simulink model "ZynqBallTrackerFPGA"  (R2017a)
settings: Solver=FixedStepDiscrete  StartTime=0.0  StopTime=5.0  RelTol=1e-3  EnableMultiTasking=on
PostLoadFcn:
  | model_init
values from neighbouring files (symbols this model uses):
  C = 1920    [model_init.m]
  HueTarg = 150    [model_init.m]
  HueTol = 20    [model_init.m]
  Kd = 1    [model_init.m]
  KernG_hdl = reshape(KernG,[],1)    [model_init.m]
  KernR1B2_hdl = reshape(KernR1B2,[],1)    [model_init.m]
  KernR2B1_hdl = reshape(KernR2B1,[],1)    [model_init.m]
  KernRB_hdl = reshape(KernRB,[],1)    [model_init.m]
  Ki = 4    [model_init.m]
  Kp = 16    [model_init.m]
  P = polyfit(u,y,N)    [calc_gamma.m]    (also in model_init.m = calc_gamma(GammaErr,3))
  PWM_CNT = 1024e3    (= 1024000)    [model_init.m]
  R = 1080    [model_init.m]
  SatTarg = 0.38    [model_init.m]
  SatTol = 0.05    [model_init.m]
  SaturationLimit = 256    [model_init.m]
  TsFPGA = TsFr/(R*C)    (= 1.60751028807e-08)    [model_init.m]
  TsFr = 1/FrRt    (= 0.0333333333333)    [model_init.m]
  ValTarg = 170    [model_init.m]
  ValTol = 45    [model_init.m]
undefined symbols (not defined in the file or in its folder): gray, Rec, SDTV
libraries: hdlsllib x51, simulink x12, simulink_need_slupdate x10, visionconversions x2, visiontextngfix x2, visionstatistics x1, dspvision x1, visiongeotforms x1, dspsigattribs x1, dspbuff3 x1
(part 2 of 2)

== system ZynqBallTrackerFPGA/fpga_dut/BallTracker/FindCentroid/y_accum ==
  Inc : Inport
  Rst : Inport  Port=2
  En : Inport  Port=3
  Add : Sum  OutDataTypeStr=fixdt(0,ceil(log2(MaxVal)),0)  RndMeth=Zero  SaturateOnIntegerOverflow=on
  Logical Operator : Logic  Operator=OR  IconShape=distinctive  AllPortsSameDT=off  OutDataTypeStr=boolean
  Switch : Switch  Criteria=u2 ~= 0
  Unit Delay Enabled : simulink_need_slupdate/Unit Delay Enabled  vinit=fi(0,0,32,0)  tsamp=-1
      settings: SourceProductName=Simulink  SourceProductBaseCode=SL
  zero : Constant  Value=0  OutDataTypeStr=Inherit: Inherit via back propagation  SampleTime=-1
  Cnt : Outport
  wires:
  En/1 -> Logical Operator/2
  Rst/1 -> Logical Operator/1, Switch/2
  zero/1 -> Switch/1
  Add/1 -> Switch/3
  Logical Operator/1 -> Unit Delay Enabled/2
  Switch/1 -> Unit Delay Enabled/1
  Inc/1 -> Add/2  "xinc"
  Unit Delay Enabled/1 -> Add/1, Cnt/1

== system ZynqBallTrackerFPGA/fpga_dut/BallTracker/OutputMux/HuetoRGB ==
  Hue : Inport
  Gain : Gain  Gain=255/360  OutDataTypeStr=fixdt(0,8,0)  RndMeth=Zero  SaturateOnIntegerOverflow=on
      settings: AttributesFormatString=|
      | ----------
      | op:3
      | ip:1
  Y2RGB : Subsystem
  RGB : Outport
  wires:
  Hue/1 -> Gain/1
  Gain/1 -> Y2RGB/1(Y_i)
  Y2RGB/1(Video_Out) -> RGB/1

== system ZynqBallTrackerFPGA/fpga_dut/BallTracker/OutputMux/SattoRGB2 ==
  Sat : Inport
  Gain : Gain  Gain=255  OutDataTypeStr=fixdt(0,8,0)  RndMeth=Zero  SaturateOnIntegerOverflow=on
      settings: AttributesFormatString=|
      | ----------
      | op:3
      | ip:1
  Y2RGB : Subsystem
  RGB : Outport
  wires:
  Sat/1 -> Gain/1
  Gain/1 -> Y2RGB/1(Y_i)
  Y2RGB/1(Video_Out) -> RGB/1

== system ZynqBallTrackerFPGA/fpga_dut/BallTracker/OutputMux/Y2RGB ==
  Y_i : Inport
  Bit Concat : hdlsllib/HDL Operations/Bit Concat  numInputs=2
      settings: SourceProductName=HDL Coder  SourceProductBaseCode=HD
  Bit Concat1 : hdlsllib/HDL Operations/Bit Concat  numInputs=2
      settings: SourceProductName=HDL Coder  SourceProductBaseCode=HD
  Bit Concat2 : hdlsllib/HDL Operations/Bit Concat  numInputs=2
      settings: SourceProductName=HDL Coder  SourceProductBaseCode=HD
  Constant : Constant  Value=0  OutDataTypeStr=uint8  SampleTime=-1
  Video_Out : Outport  OutMin=0  OutMax=255
  wires:
  Bit Concat2/1 -> Bit Concat1/2
  Y_i/1 -> Bit Concat2/2, Bit Concat2/1, Bit Concat1/1
  Bit Concat1/1 -> Bit Concat/2
  Constant/1 -> Bit Concat/1
  Bit Concat/1 -> Video_Out/1

== system ZynqBallTrackerFPGA/fpga_dut/BallTracker/OutputMux/Y2RGB1 ==
  Y_i : Inport
  Bit Concat : hdlsllib/HDL Operations/Bit Concat  numInputs=2
      settings: SourceProductName=HDL Coder  SourceProductBaseCode=HD
  Bit Concat1 : hdlsllib/HDL Operations/Bit Concat  numInputs=2
      settings: SourceProductName=HDL Coder  SourceProductBaseCode=HD
  Bit Concat2 : hdlsllib/HDL Operations/Bit Concat  numInputs=2
      settings: SourceProductName=HDL Coder  SourceProductBaseCode=HD
  Constant : Constant  Value=0  OutDataTypeStr=uint8  SampleTime=-1
  Video_Out : Outport  OutMin=0  OutMax=255
  wires:
  Bit Concat2/1 -> Bit Concat1/2
  Y_i/1 -> Bit Concat2/2, Bit Concat2/1, Bit Concat1/1
  Bit Concat1/1 -> Bit Concat/2
  Constant/1 -> Bit Concat/1
  Bit Concat/1 -> Video_Out/1

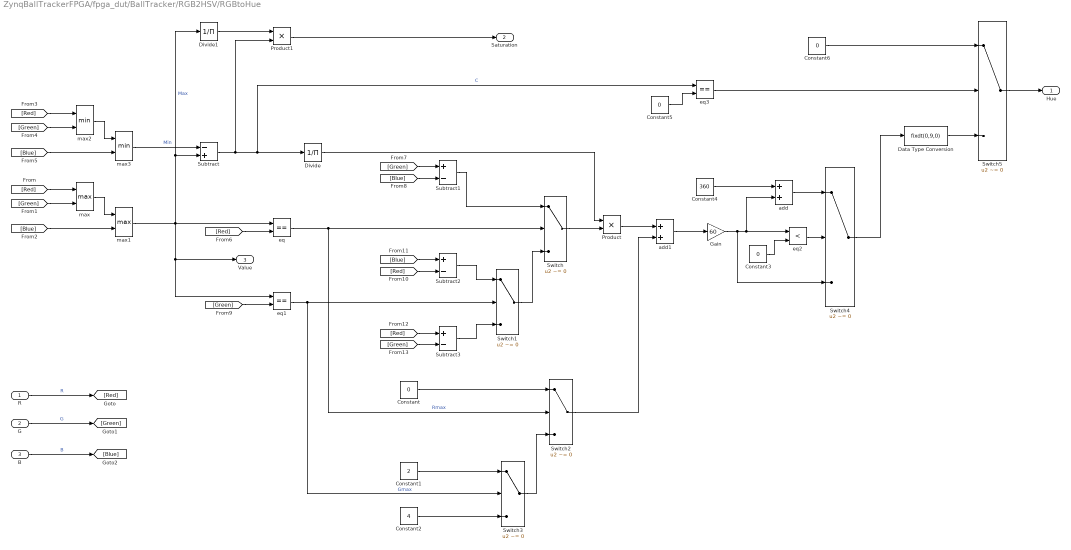
== system ZynqBallTrackerFPGA/fpga_dut/BallTracker/RGB2HSV/RGBtoHue ==
  R : Inport
  G : Inport  Port=2
  B : Inport  Port=3
  Constant : Constant  Value=0  OutDataTypeStr=fixdt(0,3,0)  SampleTime=-1
  Constant1 : Constant  Value=2  OutDataTypeStr=fixdt(0,3,0)  SampleTime=-1
  Constant2 : Constant  Value=4  OutDataTypeStr=fixdt(0,3,0)  SampleTime=-1
  Constant3 : Constant  Value=0  OutDataTypeStr=Inherit: Inherit via back propagation  SampleTime=-1
  Constant4 : Constant  Value=360  OutDataTypeStr=Inherit: Inherit via back propagation  SampleTime=-1
  Constant5 : Constant  Value=0  OutDataTypeStr=Inherit: Inherit via back propagation  SampleTime=-1
  Constant6 : Constant  Value=0  OutDataTypeStr=Inherit: Inherit via back propagation  SampleTime=-1
  Data Type Conversion : DataTypeConversion  OutDataTypeStr=fixdt(0,9,0)
  Divide : Product  Inputs=/  OutMin=1/255  OutMax=1  OutDataTypeStr=fixdt(1,16)  SaturateOnIntegerOverflow=on  RndMeth=Zero
      settings: AttributesFormatString=|
      | ----------
      | op:3
      | ip:1
  Divide1 : Product  Inputs=/  OutMin=1/255  OutMax=1  OutDataTypeStr=fixdt(0,16)  SaturateOnIntegerOverflow=on  RndMeth=Zero
      settings: AttributesFormatString=|
      | ----------
      | op:3
      | ip:1
  Gain : Gain  Gain=60  ParamDataTypeStr=fixdt(1,7)  OutDataTypeStr=fixdt(1,10,0)  RndMeth=Zero
      settings: AttributesFormatString=|
      | ----------
      | op:3
      | ip:1
  Product : Product
      settings: AttributesFormatString=|
      | ----------
      | op:3
      | ip:1
  Product1 : Product  OutDataTypeStr=fixdt(0,16,15)  SaturateOnIntegerOverflow=on  RndMeth=Zero
      settings: AttributesFormatString=|
      | ----------
      | op:3
      | ip:1
  Subtract : Sum  Inputs=-+  RndMeth=Zero  OutDataTypeStr=Inherit: Same as first input
      settings: AttributesFormatString=|
      | ----------
      | op:1
  Subtract1 : Sum  Inputs=+-  RndMeth=Zero
      settings: AttributesFormatString=|
      | ----------
      | op:1
  Subtract2 : Sum  Inputs=+-  RndMeth=Zero
      settings: AttributesFormatString=|
      | ----------
      | op:1
  Subtract3 : Sum  Inputs=+-  RndMeth=Zero
      settings: AttributesFormatString=|
      | ----------
      | op:1
  Switch{,1..5} (6 alike) : Switch  Criteria=u2 ~= 0
      settings: AttributesFormatString=|
      | ----------
      | op:1
      | ip:1
  add : Sum  OutDataTypeStr=Inherit: Inherit via back propagation  RndMeth=Zero
      settings: AttributesFormatString=|
      | ----------
      | op:1
  add1 : Sum  RndMeth=Zero  OutDataTypeStr=Inherit: Same as first input
      settings: AttributesFormatString=|
      | ----------
      | op:1
  eq : RelationalOperator  Operator===  OutDataTypeStr=boolean  RndMeth=Nearest
  eq1 : RelationalOperator  Operator===  OutDataTypeStr=boolean  RndMeth=Nearest
  eq2 : RelationalOperator  Operator=<  OutDataTypeStr=boolean  RndMeth=Nearest
  eq3 : RelationalOperator  Operator===  OutDataTypeStr=boolean  RndMeth=Nearest
  max : MinMax  Function=max  Inputs=2
  max1 : MinMax  Function=max  Inputs=2
  max2 : MinMax  Inputs=2
  max3 : MinMax  Inputs=2
  Hue : Outport
  Saturation : Outport  Port=2
  Value : Outport  Port=3
  wires:
  R/1 -> [Red]  "R"
  B/1 -> [Blue]  "B"
  G/1 -> [Green]  "G"
  [Red] -> max/1
  [Green] -> max/2
  max/1 -> max1/1
  [Blue] -> max1/2
  [Red] -> max2/1
  [Green] -> max2/2
  max2/1 -> max3/1
  [Blue] -> max3/2
  max1/1 -> eq/1, Value/1, eq1/1, Divide1/1, Subtract/2  "Max"
  max3/1 -> Subtract/1  "Min"
  [Red] -> eq/2
  [Blue] -> Subtract1/2
  [Green] -> Subtract1/1
  Switch1/1 -> Switch/3
  [Green] -> eq1/2
  eq1/1 -> Switch3/2, Switch1/2  "Gmax"
  [Blue] -> Subtract2/1
  [Red] -> Subtract2/2
  Subtract2/1 -> Switch1/1
  Subtract3/1 -> Switch1/3
  [Red] -> Subtract3/1
  [Green] -> Subtract3/2
  Subtract1/1 -> Switch/1
  Product/1 -> add1/1
  eq/1 -> Switch/2, Switch2/2  "Rmax"
  Switch/1 -> Product/2
  Subtract/1 -> Product1/2, eq3/1, Divide/1  "C"
  Divide/1 -> Product/1
  Switch3/1 -> Switch2/3
  Constant/1 -> Switch2/1
  Constant1/1 -> Switch3/1
  Constant2/1 -> Switch3/3
  Switch2/1 -> add1/2
  add1/1 -> Gain/1
  Gain/1 -> Switch4/3, add/2, eq2/1
  Constant3/1 -> eq2/2
  eq2/1 -> Switch4/2
  Constant4/1 -> add/1
  add/1 -> Switch4/1
  Constant5/1 -> eq3/2
  eq3/1 -> Switch5/2
  Switch5/1 -> Hue/1
  Switch4/1 -> Data Type Conversion/1
  Constant6/1 -> Switch5/1
  Data Type Conversion/1 -> Switch5/3
  Divide1/1 -> Product1/1
  Product1/1 -> Saturation/1

== system ZynqBallTrackerFPGA/fpga_dut/CFA/MW_CFA/Bayer_to_Vid ==
  SoF : Inport
  Bayer : Inport  Port=2
  Bit Concat{,1..3} (4 alike) : hdlsllib/HDL Operations/Bit Concat  numInputs=2
      settings: SourceProductName=HDL Coder  SourceProductBaseCode=HD
  Constant : Constant  Value=0  OutDataTypeStr=fixdt(0,7,0)  SampleTime=-1
  Video_o : Outport
  wires:
  Bit Concat1/1 -> Bit Concat3/2
  SoF/1 -> Bit Concat/1
  Bayer/1 -> Bit Concat1/1, Bit Concat2/1, Bit Concat2/2
  Bit Concat2/1 -> Bit Concat1/2
  Bit Concat/1 -> Video_o/1
  Constant/1 -> Bit Concat3/1
  Bit Concat3/1 -> Bit Concat/2

== system ZynqBallTrackerFPGA/fpga_dut/CFA/MW_CFA/Buff_5x5 ==
  Pixel : Inport
  Delay{1..4} (4 alike) : Delay  DelayLength=1  InitialCondition=0  UseCircularBuffer=on
  Integer Delay{1..4} (4 alike) : Delay  DelayLength=C
  Matrix Concatenation 25_1 : Concatenate  NumInputs=5  Mode=Multidimensional array
  Matrix Concatenation 5_1 : Concatenate  NumInputs=5  Mode=Multidimensional array
  Dly_5x5 : Outport
  wires:
  Delay2/1 -> Matrix Concatenation 25_1/2, Delay3/1
  Matrix Concatenation 5_1/1 -> Delay4/1, Matrix Concatenation 25_1/5
  Delay3/1 -> Matrix Concatenation 25_1/1
  Matrix Concatenation 25_1/1 -> Dly_5x5/1
  Delay1/1 -> Matrix Concatenation 25_1/3, Delay2/1
  Delay4/1 -> Delay1/1, Matrix Concatenation 25_1/4
  Pixel/1 -> Matrix Concatenation 5_1/5, Integer Delay1/1
  Integer Delay1/1 -> Matrix Concatenation 5_1/4, Integer Delay2/1
  Integer Delay2/1 -> Matrix Concatenation 5_1/3, Integer Delay3/1
  Integer Delay3/1 -> Matrix Concatenation 5_1/2, Integer Delay4/1
  Integer Delay4/1 -> Matrix Concatenation 5_1/1

== system ZynqBallTrackerFPGA/fpga_dut/CFA/MW_CFA/Calc_Kern ==
  Dly_5x5 : Inport
  KernG : Gain  Gain=KernG_hdl  ParamDataTypeStr=fixdt(1,8)
      settings: AttributesFormatString=|
      | ----------
      | op:3
      | ip:2
  KernR1B2 : Gain  Gain=KernR1B2_hdl  ParamDataTypeStr=fixdt(1,8)
      settings: AttributesFormatString=|
      | ----------
      | op:3
      | ip:2
  KernR2B1 : Gain  Gain=KernR2B1_hdl  ParamDataTypeStr=fixdt(1,8)
      settings: AttributesFormatString=|
      | ----------
      | op:3
      | ip:2
  KernRB : Gain  Gain=KernRB_hdl  ParamDataTypeStr=fixdt(1,8)
      settings: AttributesFormatString=|
      | ----------
      | op:3
      | ip:2
  SumG : Sum  Inputs=+  OutDataTypeStr=uint8  RndMeth=Zero  SaturateOnIntegerOverflow=on
      settings: AttributesFormatString=|
      | ----------
      | op:4
      | ip:2
  SumR1B2 : Sum  Inputs=+  OutDataTypeStr=uint8  RndMeth=Zero  SaturateOnIntegerOverflow=on
      settings: AttributesFormatString=|
      | ----------
      | op:4
      | ip:2
  SumR2B1 : Sum  Inputs=+  OutDataTypeStr=uint8  RndMeth=Zero  SaturateOnIntegerOverflow=on
      settings: AttributesFormatString=|
      | ----------
      | op:4
      | ip:2
  SumRB : Sum  Inputs=+  OutDataTypeStr=uint8  RndMeth=Zero  SaturateOnIntegerOverflow=on
      settings: AttributesFormatString=|
      | ----------
      | op:4
      | ip:2
  Ir1b2 : Outport
  Ir2b1 : Outport  Port=2
  Irb : Outport  Port=3
  Ig : Outport  Port=4
  wires:
  Dly_5x5/1 -> KernR1B2/1, KernR2B1/1, KernG/1, KernRB/1
  KernG/1 -> SumG/1
  SumR1B2/1 -> Ir1b2/1  "Ir1b2"
  SumR2B1/1 -> Ir2b1/1  "Ir2b1"
  KernRB/1 -> SumRB/1
  KernR2B1/1 -> SumR2B1/1
  SumG/1 -> Ig/1  "Ig"
  SumRB/1 -> Irb/1  "Irb"
  KernR1B2/1 -> SumR1B2/1

== system ZynqBallTrackerFPGA/fpga_dut/CFA/MW_CFA/RGB_to_Vid ==
  SoF : Inport
  R : Inport  Port=2
  G : Inport  Port=3
  B : Inport  Port=4
  Bit Concat{,1..3} (4 alike) : hdlsllib/HDL Operations/Bit Concat  numInputs=2
      settings: SourceProductName=HDL Coder  SourceProductBaseCode=HD
  Constant : Constant  Value=0  OutDataTypeStr=fixdt(0,7,0)  SampleTime=-1
  Video_o : Outport
  wires:
  Bit Concat1/1 -> Bit Concat3/2
  SoF/1 -> Bit Concat/1
  R/1 -> Bit Concat1/1
  B/1 -> Bit Concat2/2
  G/1 -> Bit Concat2/1
  Bit Concat2/1 -> Bit Concat1/2
  Bit Concat/1 -> Video_o/1
  Constant/1 -> Bit Concat3/1
  Bit Concat3/1 -> Bit Concat/2

== system ZynqBallTrackerFPGA/fpga_dut/CFA/MW_CFA/Select_Pixel ==
  note: State Encoding [RGGB]:
      | 	0 = Blue Pixel
      | 	1 = Green Pixel on blue row (1)
      | 	2 = Green Pixel on red row (2)
      | 	3 = Red Pixel
  I : Inport
  Ir1b2 : Inport  Port=2
  Ir2b1 : Inport  Port=3
  Irb : Inport  Port=4
  Ig : Inport  Port=5
  State : Inport  Port=6
  SelectBlue : Subsystem
  SelectGreen : Subsystem
  SelectRed : Subsystem
  R : Outport
  G : Outport  Port=2
  B : Outport  Port=3
  wires:
  SelectBlue/1(B) -> B/1
  SelectRed/1(R) -> R/1
  Ig/1 -> SelectGreen/2(Ig)
  I/1 -> SelectGreen/1(I), SelectBlue/1(I), SelectRed/1(I)
  Ir1b2/1 -> SelectBlue/2(Ir1b2), SelectRed/2(Ir1b2)
  State/1 -> SelectRed/5(State), SelectBlue/5(State), SelectGreen/3(State)
  Irb/1 -> SelectRed/4(Irb), SelectBlue/4(Irb)
  Ir2b1/1 -> SelectBlue/3(Ir2b1), SelectRed/3(Ir2b1)
  SelectGreen/1(G) -> G/1

== system ZynqBallTrackerFPGA/fpga_dut/CFA/MW_CFA/StateTracking ==
  Rst : Inport
  Bayer_Phase : Inport  Port=2
  Pix_Pos : Subsystem
  en : Constant  Value=true  SampleTime=-1
  state_xor : simulink/Logic and Bit Operations/Bitwise Operator  logicop=XOR  UseBitMask=off  NumInputPorts=2  BitMask=bin2dec('11011001')  BitMaskRealWorld=Stored Integer
      settings: AttributesFormatString=|
      | ----------
      | op:1
      | ip:1
  xy_to_state : Subsystem
  state : Outport
  wires:
  Rst/1 -> Pix_Pos/2(Rst)
  en/1 -> Pix_Pos/1(Vld)
  Pix_Pos/1(Column) -> xy_to_state/1(x)
  Pix_Pos/2(Row) -> xy_to_state/2(y)
  xy_to_state/1(state) -> state_xor/1
  state_xor/1 -> state/1
  Bayer_Phase/1 -> state_xor/2

== system ZynqBallTrackerFPGA/fpga_dut/CFA/MW_CFA/get_sof ==
  Video_i : Inport
  Bit Slice : hdlsllib/HDL Operations/Bit Slice  lidx=31  ridx=31
      settings: SourceProductName=HDL Coder  SourceProductBaseCode=HD
  Data Type Conversion : DataTypeConversion  OutDataTypeStr=boolean
  Delay1 : Delay  DelayLength=1
  Delay2 : Delay  DelayLength=1
  SoF : Outport
  Video_o : Outport  Port=2
  Rst : Outport  Port=3
  wires:
  Bit Slice/1 -> Data Type Conversion/1
  Video_i/1 -> Delay2/1, Bit Slice/1
  Data Type Conversion/1 -> Rst/1, Delay1/1
  Delay2/1 -> Video_o/1
  Delay1/1 -> SoF/1

== system ZynqBallTrackerFPGA/fpga_dut/GammaCorrection/Gama CorrectionCore/GammaApprox ==
  Y_i : Inport
  P : Inport  Port=2
  Data Type Conversion : DataTypeConversion  OutDataTypeStr=fixdt(0,8,8)  SaturateOnIntegerOverflow=on  RndMeth=Zero
      settings: AttributesFormatString=|
      | ----------
      | op:1
      | ip:1
  Demux : Demux
  Gain1 : Gain  Gain=256  OutDataTypeStr=fixdt(0,8,0)  RndMeth=Zero  SaturateOnIntegerOverflow=on
      settings: AttributesFormatString=|
      | ----------
      | op:1
      | ip:1
  Gain2 : Gain  Gain=1/256  OutDataTypeStr=fixdt(0,8,8)  RndMeth=Zero  SaturateOnIntegerOverflow=on
      settings: AttributesFormatString=|
      | ----------
      | op:1
      | ip:1
  Product : Product  OutDataTypeStr=fixdt(1,18,17)
      settings: AttributesFormatString=|
      | ----------
      | op:2
      | ip:1
  Product1 : Product  OutDataTypeStr=fixdt(1,18,17)  SaturateOnIntegerOverflow=on  RndMeth=Zero
      settings: AttributesFormatString=|
      | ----------
      | op:3
      | ip:1
  aDSP48E1 : Subsystem
  bDSP48E1 : Subsystem
  cDSP48E1 : Subsystem
  Y_o : Outport
  wires:
  Gain1/1 -> Y_o/1
  Y_i/1 -> Gain2/1
  P/1 -> Demux/1
  Demux/2 -> bDSP48E1/2(A)
  Demux/1 -> aDSP48E1/2(A)
  Product1/1 -> aDSP48E1/1(B)  "X3"
  Gain2/1 -> Product/1, Product/2, cDSP48E1/1(B), Product1/2  "X"
  Product/1 -> bDSP48E1/1(B), Product1/1  "X2"
  Demux/4 -> cDSP48E1/3(C)
  Demux/3 -> cDSP48E1/2(A)
  bDSP48E1/1(P) -> aDSP48E1/3(C)
  cDSP48E1/1(P) -> bDSP48E1/3(C)
  aDSP48E1/1(P) -> Data Type Conversion/1
  Data Type Conversion/1 -> Gain1/1

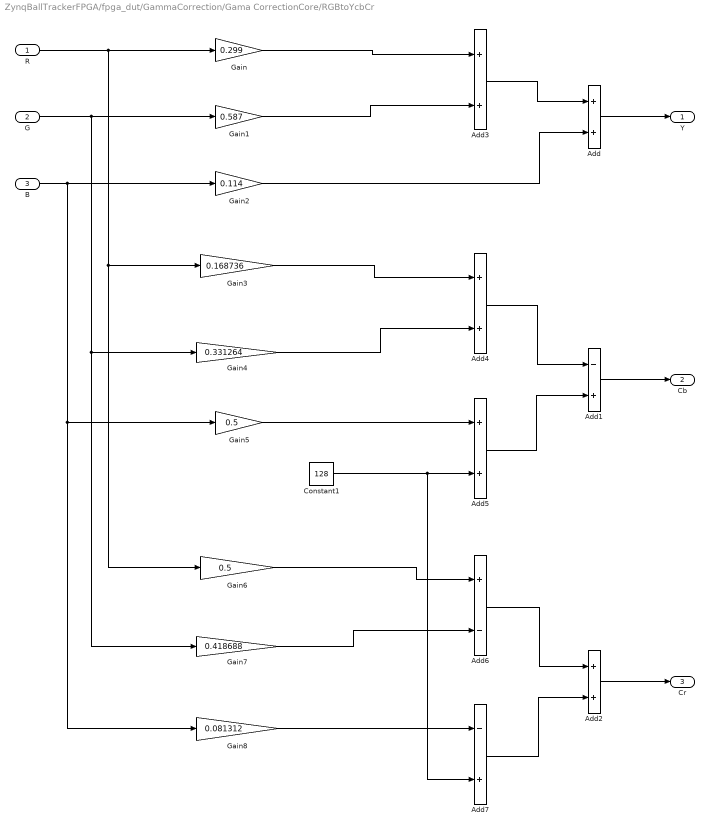
== system ZynqBallTrackerFPGA/fpga_dut/GammaCorrection/Gama CorrectionCore/RGBtoYcbCr ==
  R : Inport
  G : Inport  Port=2
  B : Inport  Port=3
  Add : Sum  OutDataTypeStr=uint8  RndMeth=Zero  SaturateOnIntegerOverflow=on
      settings: AttributesFormatString=|
      | ----------
      | op:2
      | ip:1
  Add1 : Sum  Inputs=-+  OutDataTypeStr=uint8  RndMeth=Zero  SaturateOnIntegerOverflow=on
      settings: AttributesFormatString=|
      | ----------
      | op:2
      | ip:1
  Add2 : Sum  OutDataTypeStr=uint8  RndMeth=Zero  SaturateOnIntegerOverflow=on
      settings: AttributesFormatString=|
      | ----------
      | op:2
      | ip:1
  Add3 : Sum  RndMeth=Zero  SaturateOnIntegerOverflow=on
      settings: AttributesFormatString=|
      | ----------
      | op:1
      | ip:1
  Add4 : Sum  RndMeth=Zero  SaturateOnIntegerOverflow=on
      settings: AttributesFormatString=|
      | ----------
      | op:1
      | ip:1
  Add5 : Sum  RndMeth=Zero  SaturateOnIntegerOverflow=on
      settings: AttributesFormatString=|
      | ----------
      | op:1
      | ip:1
  Add6 : Sum  Inputs=+-  RndMeth=Zero  SaturateOnIntegerOverflow=on
      settings: AttributesFormatString=|
      | ----------
      | op:1
      | ip:1
  Add7 : Sum  Inputs=-+  RndMeth=Zero  SaturateOnIntegerOverflow=on
      settings: AttributesFormatString=|
      | ----------
      | op:1
      | ip:1
  Constant1 : Constant  Value=128  OutDataTypeStr=fixdt(0,1)  SampleTime=-1
  Gain : Gain  Gain=0.299
      settings: AttributesFormatString=|
      | ----------
      | op:2
      | ip:1
  Gain1 : Gain  Gain=0.587
      settings: AttributesFormatString=|
      | ----------
      | op:2
      | ip:1
  Gain2 : Gain  Gain=0.114
      settings: AttributesFormatString=|
      | ----------
      | op:2
      | ip:1
  Gain3 : Gain  Gain=0.168736
      settings: AttributesFormatString=|
      | ----------
      | op:2
      | ip:1
  Gain4 : Gain  Gain=0.331264
      settings: AttributesFormatString=|
      | ----------
      | op:2
      | ip:1
  Gain5 : Gain  Gain=0.5
      settings: AttributesFormatString=|
      | ----------
      | op:2
      | ip:1
  Gain6 : Gain  Gain=0.5
      settings: AttributesFormatString=|
      | ----------
      | op:2
      | ip:1
  Gain7 : Gain  Gain=0.418688
      settings: AttributesFormatString=|
      | ----------
      | op:2
      | ip:1
  Gain8 : Gain  Gain=0.081312
      settings: AttributesFormatString=|
      | ----------
      | op:2
      | ip:1
  Y : Outport
  Cb : Outport  Port=2
  Cr : Outport  Port=3
  wires:
  G/1 -> Gain7/1, Gain4/1, Gain1/1
  Add/1 -> Y/1
  B/1 -> Gain8/1, Gain5/1, Gain2/1
  Constant1/1 -> Add7/2, Add5/2
  Gain3/1 -> Add4/1
  Gain5/1 -> Add5/1
  Add1/1 -> Cb/1
  R/1 -> Gain6/1, Gain3/1, Gain/1
  Gain4/1 -> Add4/2
  Gain6/1 -> Add6/1
  Gain8/1 -> Add7/1
  Add2/1 -> Cr/1
  Gain7/1 -> Add6/2
  Gain1/1 -> Add3/2
  Gain2/1 -> Add/2
  Gain/1 -> Add3/1
  Add3/1 -> Add/1
  Add4/1 -> Add1/1
  Add5/1 -> Add1/2
  Add6/1 -> Add2/1
  Add7/1 -> Add2/2

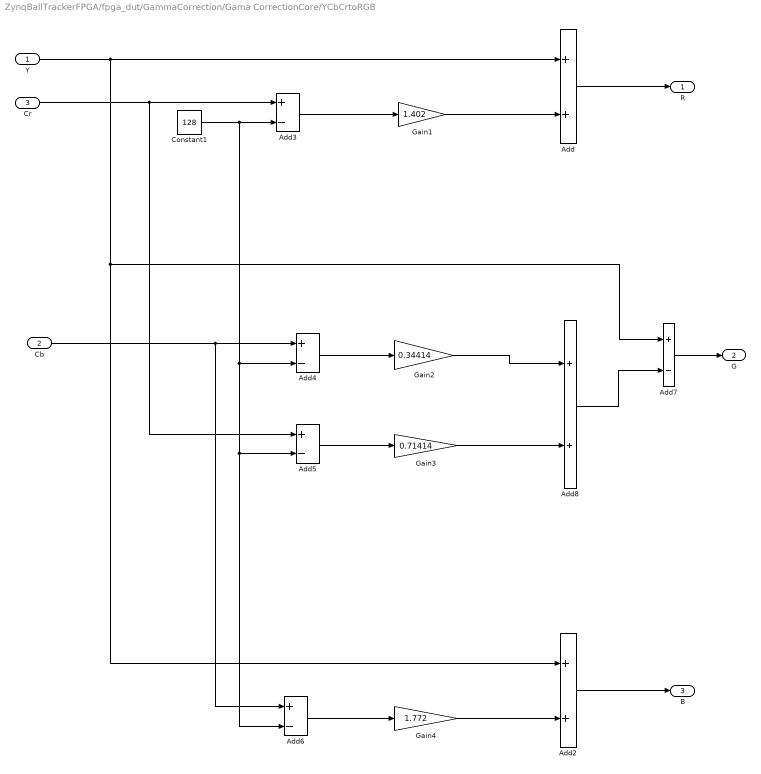
== system ZynqBallTrackerFPGA/fpga_dut/GammaCorrection/Gama CorrectionCore/YCbCrtoRGB ==
  Y : Inport
  Cb : Inport  Port=2
  Cr : Inport  Port=3
  Add : Sum  Inputs=2  OutDataTypeStr=uint8  RndMeth=Zero  SaturateOnIntegerOverflow=on
      settings: AttributesFormatString=|
      | ----------
      | op:2
      | ip:1
  Add2 : Sum  Inputs=2  OutDataTypeStr=uint8  RndMeth=Zero  SaturateOnIntegerOverflow=on
      settings: AttributesFormatString=|
      | ----------
      | op:2
      | ip:1
  Add{3..6} (4 alike) : Sum  Inputs=+-  RndMeth=Zero
      settings: AttributesFormatString=|
      | ----------
      | op:1
      | ip:1
  Add7 : Sum  Inputs=+-  OutDataTypeStr=uint8  RndMeth=Zero  SaturateOnIntegerOverflow=on
      settings: AttributesFormatString=|
      | ----------
      | op:2
      | ip:1
  Add8 : Sum  RndMeth=Zero  SaturateOnIntegerOverflow=on
      settings: AttributesFormatString=|
      | ----------
      | op:1
      | ip:1
  Constant1 : Constant  Value=128  OutDataTypeStr=fixdt(0,1)  SampleTime=-1
  Gain1 : Gain  Gain=1.402
      settings: AttributesFormatString=|
      | ----------
      | op:2
      | ip:1
  Gain2 : Gain  Gain=0.34414
      settings: AttributesFormatString=|
      | ----------
      | op:2
      | ip:1
  Gain3 : Gain  Gain=0.71414
      settings: AttributesFormatString=|
      | ----------
      | op:2
      | ip:1
  Gain4 : Gain  Gain=1.772
      settings: AttributesFormatString=|
      | ----------
      | op:2
      | ip:1
  R : Outport
  G : Outport  Port=2
  B : Outport  Port=3
  wires:
  Y/1 -> Add7/1, Add2/1, Add/1
  Add/1 -> R/1
  Cr/1 -> Add5/1, Add3/1
  Constant1/1 -> Add6/2, Add5/2, Add4/2, Add3/2
  Add3/1 -> Gain1/1
  Gain1/1 -> Add/2
  Gain3/1 -> Add8/2
  Gain2/1 -> Add8/1
  Add4/1 -> Gain2/1
  Add5/1 -> Gain3/1
  Cb/1 -> Add6/1, Add4/1
  Add2/1 -> B/1
  Add6/1 -> Gain4/1
  Gain4/1 -> Add2/2
  Add7/1 -> G/1
  Add8/1 -> Add7/2

== system ZynqBallTrackerFPGA/fpga_dut/motor_ctl/ADC_DUT/Debounce ==
  In : Inport
  Chart : Stateflow chart  TreatAsAtomicUnit=on
  Constant : Constant  Value=debounce_count  OutDataTypeStr=uint8  SampleTime=-1
  Out : Outport
  wires:
  Constant/1 -> Chart/2(count_debounce)
  Chart/1(y) -> Out/1
  In/1 -> Chart/1(u)

== system ZynqBallTrackerFPGA/fpga_dut/motor_ctl/ADC_DUT/reduce_8_to_4 ==
  In1 : Inport
  Bit Concat : hdlsllib/HDL Operations/Bit Concat  numInputs=4
      settings: SourceProductName=HDL Coder  SourceProductBaseCode=HD
  Bit Slice : hdlsllib/HDL Operations/Bit Slice  lidx=1  ridx=1
      settings: SourceProductName=HDL Coder  SourceProductBaseCode=HD
  Bit Slice1 : hdlsllib/HDL Operations/Bit Slice  lidx=3  ridx=3
      settings: SourceProductName=HDL Coder  SourceProductBaseCode=HD
  Bit Slice2 : hdlsllib/HDL Operations/Bit Slice  lidx=5  ridx=5
      settings: SourceProductName=HDL Coder  SourceProductBaseCode=HD
  Bit Slice3 : hdlsllib/HDL Operations/Bit Slice  lidx=7  ridx=7
      settings: SourceProductName=HDL Coder  SourceProductBaseCode=HD
  Out1 : Outport
  wires:
  Bit Slice/1 -> Bit Concat/4
  Bit Slice1/1 -> Bit Concat/3
  Bit Slice2/1 -> Bit Concat/2
  Bit Slice3/1 -> Bit Concat/1
  Bit Concat/1 -> Out1/1
  In1/1 -> Bit Slice2/1, Bit Slice1/1, Bit Slice/1, Bit Slice3/1

== system ZynqBallTrackerFPGA/fpga_dut/motor_ctl/PID_Controller/PID_Controller_Programmable ==
  error_delta : Inport
  PGain : Inport  Port=2  LockScale=on
  IGain : Inport  Port=3
  DGain : Inport  Port=4  LockScale=on
  Controller : Subsystem  MinMaxOverflowLogging=MinMaxAndOverflow
  InputRegister{1..4} (4 alike) : Delay  DelayLength=1  InputProcessing=Inherited
  OutputRegister1 : Delay  DelayLength=1  InputProcessing=Inherited
  controlsignal : Outport
  wires:
  OutputRegister1/1 -> controlsignal/1
  InputRegister1/1 -> Controller/1(error_delta)
  InputRegister3/1 -> Controller/4(Dgain)
  InputRegister2/1 -> Controller/2(Pgain)
  IGain/1 -> InputRegister4/1  "sdo_igain"
  DGain/1 -> InputRegister3/1  "sdo_dgain"
  PGain/1 -> InputRegister2/1  "sdo_pgain"
  error_delta/1 -> InputRegister1/1
  Controller/1(controlsignal) -> OutputRegister1/1
  InputRegister4/1 -> Controller/3(Igain)

== system ZynqBallTrackerFPGA/fpga_dut/motor_ctl/pwm_controller/pwm_bist ==
  drive_p_in : Inport
  drive_n_in : Inport  Port=2
  force_p : Inport  Port=3
  force_n : Inport  Port=4
  disable : Inport  Port=5
  Logical Operator1 : Logic  Operator=NOT  IconShape=distinctive  AllPortsSameDT=off  OutDataTypeStr=boolean
  Logical Operator{3,7,9..10} (4 alike) : Logic  Inputs=3  IconShape=distinctive  AllPortsSameDT=off  OutDataTypeStr=boolean
  Logical Operator2 : Logic  Operator=OR  IconShape=distinctive  AllPortsSameDT=off  OutDataTypeStr=boolean
  Logical Operator4 : Logic  Operator=NAND  Inputs=3  IconShape=distinctive  AllPortsSameDT=off  OutDataTypeStr=boolean
  Logical Operator5 : Logic  Operator=OR  IconShape=distinctive  AllPortsSameDT=off  OutDataTypeStr=boolean
  Logical Operator6 : Logic  Operator=NOT  IconShape=distinctive  AllPortsSameDT=off  OutDataTypeStr=boolean
  Logical Operator8 : Logic  Operator=NOT  IconShape=distinctive  AllPortsSameDT=off  OutDataTypeStr=boolean
  drive_p_out : Outport
  drive_n_out : Outport  Port=2
  reset_cntr : Outport  Port=3
  wires:
  disable/1 -> Logical Operator1/1
  Logical Operator4/1 -> reset_cntr/1
  Logical Operator1/1 -> Logical Operator3/2, Logical Operator7/2, Logical Operator10/3, Logical Operator9/3, Logical Operator4/3
  force_n/1 -> Logical Operator3/3, Logical Operator8/1
  force_p/1 -> Logical Operator7/3, Logical Operator6/1
  Logical Operator10/1 -> Logical Operator5/1
  Logical Operator9/1 -> Logical Operator2/1
  Logical Operator7/1 -> Logical Operator2/2
  Logical Operator3/1 -> Logical Operator5/2
  Logical Operator2/1 -> drive_p_out/1
  Logical Operator5/1 -> drive_n_out/1
  drive_p_in/1 -> Logical Operator9/1
  drive_n_in/1 -> Logical Operator10/1
  Logical Operator6/1 -> Logical Operator4/1, Logical Operator10/2, Logical Operator3/1
  Logical Operator8/1 -> Logical Operator4/2, Logical Operator9/2, Logical Operator7/1

== system ZynqBallTrackerFPGA/fpga_dut/motor_ctl/pwm_controller/pwm_logic ==
  note: At the end of every period
      | latch the value for duty-cycle
      | and the direction
  inref : Inport
  polarity : Inport  Port=2
  reset : Inport  Port=3
  pwm_cnt : Inport  Port=4
  Bit Shift : hdlsllib/HDL Operations/Bit Shift  mode=Shift Right Arithmetic  N=8
      settings: SourceProductName=HDL Coder  SourceProductBaseCode=HD
  HDL Counter : hdlsllib/HDL Operations/HDL Counter  CountType=Free running  CountInit=0  CountStep=1  CountMax=10e5  CountFromType=Initial value  CountFrom=0  CountResetPort=on  CountLoadPort=off  CountEnbPort=off  CountDirPort=off  CountDataType=Unsigned  CountWordLen=22  CountFracLen=0  CountSampTime=-1
      settings: SourceProductName=HDL Coder  SourceProductBaseCode=HD
  Logical Operator : Logic  Inputs=3  IconShape=distinctive  AllPortsSameDT=off  OutDataTypeStr=boolean
  Logical Operator1 : Logic  Inputs=3  IconShape=distinctive  AllPortsSameDT=off  OutDataTypeStr=boolean
  Logical Operator2 : Logic  Operator=NOT  IconShape=distinctive  AllPortsSameDT=off  OutDataTypeStr=boolean
  Logical Operator3 : Logic  Operator=NOT  IconShape=distinctive  AllPortsSameDT=off  OutDataTypeStr=boolean
  Logical Operator4 : Logic  Operator=OR  IconShape=distinctive  AllPortsSameDT=off  OutDataTypeStr=boolean
  Product : Product
  Relational Operator : RelationalOperator  Operator=<  OutDataTypeStr=boolean  RndMeth=Nearest
  Relational Operator1 : RelationalOperator  OutDataTypeStr=boolean  RndMeth=Nearest
  Unit Delay Enabled : simulink_need_slupdate/Unit Delay Enabled  vinit=0.0  tsamp=-1
      settings: SourceProductName=Simulink  SourceProductBaseCode=SL
  Unit Delay Enabled1 : simulink_need_slupdate/Unit Delay Enabled  vinit=0.0  tsamp=-1
      settings: SourceProductName=Simulink  SourceProductBaseCode=SL
  drive_p : Outport
  drive_n : Outport  Port=2
  pwm_trig : Outport  Port=3
  wires:
  Unit Delay Enabled1/1 -> Logical Operator/2, Logical Operator3/1
  reset/1 -> Logical Operator2/1, Logical Operator4/1
  Logical Operator2/1 -> Logical Operator1/3, Logical Operator/3
  Relational Operator1/1 -> pwm_trig/1, Unit Delay Enabled1/2, Logical Operator4/2, Unit Delay Enabled/2
  polarity/1 -> Unit Delay Enabled1/1
  Logical Operator1/1 -> drive_n/1
  inref/1 -> Unit Delay Enabled/1
  Logical Operator/1 -> drive_p/1
  Relational Operator/1 -> Logical Operator1/1, Logical Operator/1
  HDL Counter/1 -> Relational Operator1/1, Relational Operator/1
  Unit Delay Enabled/1 -> Product/1
  Product/1 -> Relational Operator/2
  pwm_cnt/1 -> Relational Operator1/2, Bit Shift/1
  Logical Operator4/1 -> HDL Counter/1
  Bit Shift/1 -> Product/2
  Logical Operator3/1 -> Logical Operator1/2

== system ZynqBallTrackerFPGA/fpga_dut/BallTracker/FindCentroid/TimingSubsystem/Pix_Pos ==
  Vld : Inport
  Rst : Inport  Port=2
  ColLimit : simulink/Logic and Bit Operations/Compare To Constant  relop===  const=C-1  OutDataTypeStr=boolean
  ColumnCntr : hdlsllib/HDL Operations/HDL Counter  CountType=Count limited  CountInit=0  CountStep=1  CountMax=C-1  CountFromType=Initial value  CountFrom=0  CountResetPort=on  CountLoadPort=off  CountEnbPort=on  CountDirPort=off  CountDataType=Unsigned  CountWordLen=ceil(log2(C))  CountFracLen=0  CountSampTime=1
      settings: SourceProductName=HDL Coder  SourceProductBaseCode=HD
  Logical Operator : Logic  AllPortsSameDT=off  OutDataTypeStr=boolean
  RowCntr : hdlsllib/HDL Operations/HDL Counter  CountType=Count limited  CountInit=0  CountStep=1  CountMax=R-1  CountFromType=Initial value  CountFrom=0  CountResetPort=on  CountLoadPort=off  CountEnbPort=on  CountDirPort=off  CountDataType=Unsigned  CountWordLen=ceil(log2(R))  CountFracLen=0  CountSampTime=1
      settings: SourceProductName=HDL Coder  SourceProductBaseCode=HD
  Column : Outport
  Row : Outport  Port=2
  wires:
  Vld/1 -> Logical Operator/2, ColumnCntr/2  "enable"
  ColumnCntr/1 -> Column/1, ColLimit/1  "column"
  RowCntr/1 -> Row/1  "row"
  ColLimit/1 -> Logical Operator/1  "new_row"
  Rst/1 -> RowCntr/1, ColumnCntr/1  "rst"
  Logical Operator/1 -> RowCntr/2

== system ZynqBallTrackerFPGA/fpga_dut/BallTracker/OutputMux/HuetoRGB/Y2RGB ==
  Y_i : Inport
  Bit Concat : hdlsllib/HDL Operations/Bit Concat  numInputs=2
      settings: SourceProductName=HDL Coder  SourceProductBaseCode=HD
  Bit Concat1 : hdlsllib/HDL Operations/Bit Concat  numInputs=2
      settings: SourceProductName=HDL Coder  SourceProductBaseCode=HD
  Bit Concat2 : hdlsllib/HDL Operations/Bit Concat  numInputs=2
      settings: SourceProductName=HDL Coder  SourceProductBaseCode=HD
  Constant : Constant  Value=0  OutDataTypeStr=uint8  SampleTime=-1
  Video_Out : Outport  OutMin=0  OutMax=255
  wires:
  Bit Concat/1 -> Video_Out/1
  Constant/1 -> Bit Concat/1
  Bit Concat1/1 -> Bit Concat/2
  Y_i/1 -> Bit Concat1/1, Bit Concat2/1, Bit Concat2/2
  Bit Concat2/1 -> Bit Concat1/2

== system ZynqBallTrackerFPGA/fpga_dut/BallTracker/OutputMux/SattoRGB2/Y2RGB ==
  Y_i : Inport
  Bit Concat : hdlsllib/HDL Operations/Bit Concat  numInputs=2
      settings: SourceProductName=HDL Coder  SourceProductBaseCode=HD
  Bit Concat1 : hdlsllib/HDL Operations/Bit Concat  numInputs=2
      settings: SourceProductName=HDL Coder  SourceProductBaseCode=HD
  Bit Concat2 : hdlsllib/HDL Operations/Bit Concat  numInputs=2
      settings: SourceProductName=HDL Coder  SourceProductBaseCode=HD
  Constant : Constant  Value=0  OutDataTypeStr=uint8  SampleTime=-1
  Video_Out : Outport  OutMin=0  OutMax=255
  wires:
  Bit Concat/1 -> Video_Out/1
  Constant/1 -> Bit Concat/1
  Bit Concat1/1 -> Bit Concat/2
  Y_i/1 -> Bit Concat1/1, Bit Concat2/1, Bit Concat2/2
  Bit Concat2/1 -> Bit Concat1/2

== system ZynqBallTrackerFPGA/fpga_dut/CFA/MW_CFA/Select_Pixel/SelectBlue ==
  I : Inport
  Ir1b2 : Inport  Port=2
  Ir2b1 : Inport  Port=3
  Irb : Inport  Port=4
  State : Inport  Port=5
  Multiport Switch : MultiPortSwitch  DataPortOrder=Zero-based contiguous  Inputs=4
      settings: AttributesFormatString=|
      | ----------
      | op:1
      | ip:1
  B : Outport
  wires:
  Multiport Switch/1 -> B/1  "blue"
  State/1 -> Multiport Switch/1
  Irb/1 -> Multiport Switch/5
  I/1 -> Multiport Switch/2
  Ir1b2/1 -> Multiport Switch/4
  Ir2b1/1 -> Multiport Switch/3

== system ZynqBallTrackerFPGA/fpga_dut/CFA/MW_CFA/Select_Pixel/SelectGreen ==
  I : Inport
  Ig : Inport  Port=2
  State : Inport  Port=3
  Multiport Switch : MultiPortSwitch  DataPortOrder=Zero-based contiguous  Inputs=4
      settings: AttributesFormatString=|
      | ----------
      | op:1
      | ip:1
  G : Outport
  wires:
  I/1 -> Multiport Switch/3, Multiport Switch/4
  Ig/1 -> Multiport Switch/5, Multiport Switch/2
  Multiport Switch/1 -> G/1  "green"
  State/1 -> Multiport Switch/1

== system ZynqBallTrackerFPGA/fpga_dut/CFA/MW_CFA/Select_Pixel/SelectRed ==
  I : Inport
  Ir1b2 : Inport  Port=2
  Ir2b1 : Inport  Port=3
  Irb : Inport  Port=4
  State : Inport  Port=5
  Multiport Switch : MultiPortSwitch  DataPortOrder=Zero-based contiguous  Inputs=4
      settings: AttributesFormatString=|
      | ----------
      | op:1
      | ip:1
  R : Outport
  wires:
  State/1 -> Multiport Switch/1
  Multiport Switch/1 -> R/1  "red"
  I/1 -> Multiport Switch/5
  Irb/1 -> Multiport Switch/2
  Ir2b1/1 -> Multiport Switch/4
  Ir1b2/1 -> Multiport Switch/3

== system ZynqBallTrackerFPGA/fpga_dut/CFA/MW_CFA/StateTracking/Pix_Pos ==
  Vld : Inport
  Rst : Inport  Port=2
  ColLimit : simulink/Logic and Bit Operations/Compare To Constant  relop===  const=C-1  OutDataTypeStr=boolean
  ColumnCntr : hdlsllib/HDL Operations/HDL Counter  CountType=Count limited  CountInit=0  CountStep=1  CountMax=C-1  CountFromType=Initial value  CountFrom=0  CountResetPort=on  CountLoadPort=off  CountEnbPort=on  CountDirPort=off  CountDataType=Unsigned  CountWordLen=ceil(log2(C))  CountFracLen=0  CountSampTime=1
      settings: SourceProductName=HDL Coder  SourceProductBaseCode=HD
  Logical Operator : Logic  AllPortsSameDT=off  OutDataTypeStr=boolean
  RowCntr : hdlsllib/HDL Operations/HDL Counter  CountType=Count limited  CountInit=0  CountStep=1  CountMax=R-1  CountFromType=Initial value  CountFrom=0  CountResetPort=on  CountLoadPort=off  CountEnbPort=on  CountDirPort=off  CountDataType=Unsigned  CountWordLen=ceil(log2(R))  CountFracLen=0  CountSampTime=1
      settings: SourceProductName=HDL Coder  SourceProductBaseCode=HD
  Column : Outport
  Row : Outport  Port=2
  wires:
  Vld/1 -> Logical Operator/2, ColumnCntr/2  "enable"
  ColumnCntr/1 -> Column/1, ColLimit/1  "column"
  RowCntr/1 -> Row/1  "row"
  ColLimit/1 -> Logical Operator/1  "new_row"
  Rst/1 -> RowCntr/1, ColumnCntr/1  "rst"
  Logical Operator/1 -> RowCntr/2

== system ZynqBallTrackerFPGA/fpga_dut/CFA/MW_CFA/StateTracking/xy_to_state ==
  x : Inport
  y : Inport  Port=2
  Bit Concat : hdlsllib/HDL Operations/Bit Concat  numInputs=2
      settings: SourceProductName=HDL Coder  SourceProductBaseCode=HD
  GetLSB_x : hdlsllib/HDL Operations/Bit Slice  lidx=0  ridx=0
      settings: SourceProductName=HDL Coder  SourceProductBaseCode=HD
  GetLSB_y : hdlsllib/HDL Operations/Bit Slice  lidx=0  ridx=0
      settings: SourceProductName=HDL Coder  SourceProductBaseCode=HD
  state : Outport
  wires:
  x/1 -> GetLSB_x/1
  y/1 -> GetLSB_y/1
  Bit Concat/1 -> state/1
  GetLSB_x/1 -> Bit Concat/2
  GetLSB_y/1 -> Bit Concat/1

== system ZynqBallTrackerFPGA/fpga_dut/GammaCorrection/Gama CorrectionCore/GammaApprox/aDSP48E1 ==
  note: Implements P = B*A + C
      | 	B = 18-bit input
      | 	A = 25-bit input
      | 	C = 48-bit input
      |
      | Consumes pipeline registers of DSP48E1
  B : Inport
  A : Inport  Port=2
  C : Inport  Port=3
  adder : Sum  RndMeth=Zero
      settings: AttributesFormatString=|
      | ----------
      | op:1
      | ip:1
  mult : Product
      settings: AttributesFormatString=|
      | ----------
      | ip:1
  P : Outport
  wires:
  A/1 -> mult/2  "a"
  B/1 -> mult/1  "b"
  C/1 -> adder/2  "c_in"
  adder/1 -> P/1  "p"
  mult/1 -> adder/1  "m"

== system ZynqBallTrackerFPGA/fpga_dut/GammaCorrection/Gama CorrectionCore/GammaApprox/bDSP48E1 ==
  note: Implements P = B*A + C
      | 	B = 18-bit input
      | 	A = 25-bit input
      | 	C = 48-bit input
      |
      | Consumes pipeline registers of DSP48E1
  B : Inport
  A : Inport  Port=2
  C : Inport  Port=3
  adder : Sum  RndMeth=Zero
      settings: AttributesFormatString=|
      | ----------
      | op:1
      | ip:1
  mult : Product
      settings: AttributesFormatString=|
      | ----------
      | ip:1
  P : Outport
  wires:
  mult/1 -> adder/1  "m"
  adder/1 -> P/1  "p"
  C/1 -> adder/2  "c_in"
  B/1 -> mult/1  "b"
  A/1 -> mult/2  "a"

== system ZynqBallTrackerFPGA/fpga_dut/GammaCorrection/Gama CorrectionCore/GammaApprox/cDSP48E1 ==
  note: Implements P = B*A + C
      | 	B = 18-bit input
      | 	A = 25-bit input
      | 	C = 48-bit input
      |
      | Consumes pipeline registers of DSP48E1
  B : Inport
  A : Inport  Port=2
  C : Inport  Port=3
  adder : Sum  RndMeth=Zero
      settings: AttributesFormatString=|
      | ----------
      | op:1
      | ip:1
  mult : Product
      settings: AttributesFormatString=|
      | ----------
      | ip:1
  P : Outport
  wires:
  A/1 -> mult/2  "a"
  B/1 -> mult/1  "b"
  C/1 -> adder/2  "c_in"
  adder/1 -> P/1  "p"
  mult/1 -> adder/1  "m"

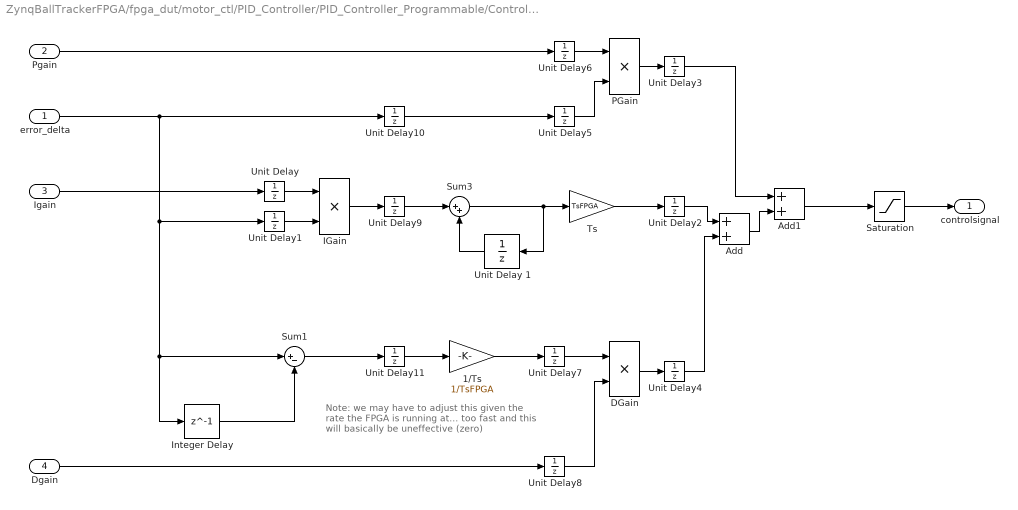
== system ZynqBallTrackerFPGA/fpga_dut/motor_ctl/PID_Controller/PID_Controller_Programmable/Controller ==
  note: Note: we may have to adjust this given
      | the rate the FPGA is running at... too fast
      | and this will basically be uneffective (zero)
  error_delta : Inport
  Pgain : Inport  Port=2
  Igain : Inport  Port=3
  Dgain : Inport  Port=4
  1/Ts : Gain  Gain=1/TsFPGA  SaturateOnIntegerOverflow=on
  Add : Sum
  Add1 : Sum
  DGain : Product  OutDataTypeStr=fixdt(1,24,0)
  IGain : Product
  Integer Delay : Delay  DelayLength=1  InputProcessing=Inherited
  PGain : Product
  Saturation : Saturate  UpperLimit=SaturationLimit-1  LowerLimit=-SaturationLimit  OutDataTypeStr=fixdt(1,9,0)
  Sum1 : Sum  Inputs=|+-  AccumDataTypeStr=fixdt(1,16,0)
  Sum3 : Sum  Inputs=|++  AccumDataTypeStr=fixdt(1,10,0)  OutDataTypeStr=fixdt(1,16,0)
  Ts : Gain  Gain=TsFPGA  SaturateOnIntegerOverflow=on
  Unit Delay{,1..11} (12 alike) : UnitDelay  SampleTime=-1
  Unit Delay 1 : UnitDelay  SampleTime=-1
  controlsignal : Outport
  wires:
  Saturation/1 -> controlsignal/1
  Dgain/1 -> Unit Delay8/1
  Pgain/1 -> Unit Delay6/1
  PGain/1 -> Unit Delay3/1
  1/Ts/1 -> Unit Delay7/1
  Sum1/1 -> Unit Delay11/1
  Integer Delay/1 -> Sum1/2
  error_delta/1 -> Unit Delay1/1, Integer Delay/1, Sum1/1, Unit Delay10/1
  DGain/1 -> Unit Delay4/1
  Sum3/1 -> Ts/1, Unit Delay 1/1
  Unit Delay 1/1 -> Sum3/2
  Igain/1 -> Unit Delay/1
  Unit Delay/1 -> IGain/1
  Unit Delay1/1 -> IGain/2
  Unit Delay2/1 -> Add/1
  Unit Delay3/1 -> Add1/1
  Unit Delay4/1 -> Add/2
  Unit Delay5/1 -> PGain/2
  Unit Delay6/1 -> PGain/1
  Unit Delay7/1 -> DGain/1
  Unit Delay8/1 -> DGain/2
  Add1/1 -> Saturation/1
  Add/1 -> Add1/2
  IGain/1 -> Unit Delay9/1
  Ts/1 -> Unit Delay2/1
  Unit Delay9/1 -> Sum3/1
  Unit Delay10/1 -> Unit Delay5/1
  Unit Delay11/1 -> 1/Ts/1

== stateflow chart ZynqBallTrackerFPGA/fpga_dut/motor_ctl/ADC_DUT/Debounce/Chart ==
  settings: executeAtInitialization=1
  (default) -> (junction 2)
  (junction 2) -> (junction 3) [order 1] : [u == u_n1]
  (junction 2) -> (junction 13) [order 2] : {count = 0;}
  (junction 3) -> (junction 5)
  (junction 5) -> (junction 7) [order 1] : [count >= count_debounce]
  (junction 7) -> (junction 9) : {y = u;}
  (junction 5) -> (junction 11) [order 2] : {count = count + 1;}
  (junction 11) -> (junction 13)
  (junction 9) -> (junction 11)
  (junction 13) -> (junction 17) : {u_n1 = u;}
  data: u input; u_n1 local type(u); y output type(u); count local uint8; count_debounce input

== matlab function ZynqBallTrackerFPGA/CameraPlant/mosaic ==
  data: I input; Y output; phase input
function Y = mosaic(I, phase)
    if(size(I,3) ~= 3)
        error('Input must be a MxNx3 matrix in RGB format');
    end
    
    phase = uint8(mod(phase,4));
    
    nrow = size(I,1);
    ncol = size(I,2);
    Y = uint8(zeros(nrow, ncol));

    for y = 1:nrow
        for x = 1:ncol
            state = uint8(mod(x-1,2) + 2*mod(y-1,2));    
            state = bitxor(state,phase);
            
            switch state % BGGR
                case 0 %B
                    Y(y,x) = I(y,x,3);
                case 1 %G
                    Y(y,x) = I(y,x,2);
                case 2 %G
                    Y(y,x) = I(y,x,2);
                case 3 %R
                    Y(y,x) = I(y,x,1);
            end
        end
    end
end

== matlab function ZynqBallTrackerFPGA/deserialize/RGB32_to_RGB ==
  data: RGB32 input; RGB output; doTranspose parameter
function RGB  = RBG32_to_RGB(RGB32, doTranspose)
if numel(RGB32) == 1
    sz = [1 1];
    RGB32_i = reshape(RGB32,sz);
    pixelMode = coder.const(true);
else
    sz = size(RGB32);
    RGB32_i = RGB32;
    pixelMode = coder.const(false);
end
nFrames = size(RGB32_i,3);
if pixelMode
    outSize = [1 3];
else
    if doTranspose
        outSize =[sz(2:-1:1) 3 nFrames];
    else
        outSize =[sz(1:2) 3 nFrames];
    end    
end
RGB = coder.nullcopy(uint8(zeros(outSize)));
for frameIdx = 1:nFrames
    if doTranspose
        RGB32_int = transpose(RGB32_i(:,:,frameIdx));
    else
        RGB32_int = RGB32_i(:,:,frameIdx);
    end
    for bitIdx = coder.unroll(0:2)
        if pixelMode
            RGB(3-bitIdx) = bitsliceget(RGB32_int,(bitIdx+1)*8,bitIdx*8+1);    
        else
            RGB(:,:,3-bitIdx,frameIdx) = bitsliceget(RGB32_int,(bitIdx+1)*8,bitIdx*8+1);    
        end
    end
end

== matlab function ZynqBallTrackerFPGA/Serialize/RGB_to_RGB32 ==
  data: RGB32 output; R input; G input; B input
function RGB32 = RBG_to_RGB32(R,G,B)
RGB32_int = uint32(zeros(size(R)));
SoF = zeros(size(R));
SoF(1,1) = hex2dec('80');
RGB32_int = set_byte(RGB32_int,SoF,24);
RGB32_int = set_byte(RGB32_int,R,16);
RGB32_int = set_byte(RGB32_int,G,8);
RGB32_int = set_byte(RGB32_int,B,0);
RGB32 = RGB32_int';

function dword = set_byte(dword,val,pos)
dword = bitor(dword,bitshift(bitand(uint32(val), hex2dec('FF')),pos));
